simulink model "Full_model_M_function_spring_stiffness"  (R2018a)
settings: Solver=VariableStepAuto  StartTime=0.0  StopTime=10.0  FixedStep=0.00000001  RelTol=1e-3
values from neighbouring files (symbols this model uses):
  bs = 2000    [suspensiondata.mat]
  bse = 3000    [suspensiondata.mat]
  Kse = 8000    [suspensiondata.mat]
  Kt = 125000    [suspensiondata.mat]
  Ms = 250    [suspensiondata.mat]
  Mse = 90    [suspensiondata.mat]
  Mu = 40    [suspensiondata.mat]
  Zr = 0.2    [suspensiondata.mat]
undefined symbols (not defined in the file or in its folder): poly_coeffs, x_data, x_pivot, y_data, ypivot
settings Model: Creator=Saurabh Suman  LastModifiedBy=Saurabh Suman

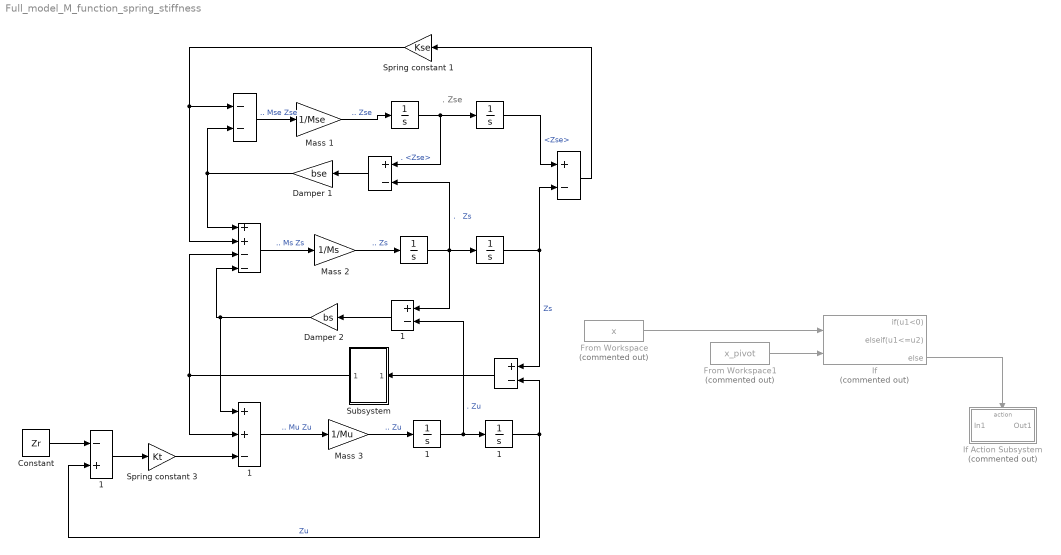
== system Full_model_M_function_spring_stiffness ==
  note: .
      | Zse
  " " : Integrator
  "  " : Sum  Inputs=+-
  "     " : Integrator
  "      " : Sum  Inputs=++--
  "       " : Sum  Inputs=--
  "        " : Sum  Inputs=+-
  "         " : Integrator
  "          " : Integrator
  "             " : Sum  Inputs=+-
  "             1" : Sum  Inputs=+-
  "          1" : Integrator
  "         1" : Integrator
  "       1" : Sum  Inputs=-+
  "      1" : Sum  Inputs=++-
  Constant : Constant  Value=Zr
  Damper 1 : Gain  Gain=bse
  Damper 2 : Gain  Gain=bs
  From Workspace : FromWorkspace  Commented=on  VariableName=x  SampleTime=0
  From Workspace1 : FromWorkspace  Commented=on  VariableName=x_pivot  SampleTime=0
  If : If  Commented=on  NumInputs=2  IfExpression=u1<0  ElseIfExpressions=u1<=u2
  If Action Subsystem : Subsystem  Commented=on  TreatAsAtomicUnit=on
  Mass 1 : Gain  Gain=1/Mse
  Mass 2 : Gain  Gain=1/Ms
  Mass 3 : Gain  Gain=1/Mu
  Spring constant 1 : Gain  Gain=Kse
  Spring constant 3 : Gain  Gain=Kt
  Subsystem : Subsystem
  wires:
  "     "/1 -> "  "/1  "<Zse>"
  "       1"/1 -> Spring constant 3/1
  " "/1 -> "        "/1, "     "/1  ". <Zse>"
  Mass 1/1 -> " "/1  ".. Zse"
  Damper 1/1 -> "      "/1, "       "/2
  Damper 2/1 -> "      "/4, "      1"/1
  Spring constant 3/1 -> "      1"/3
  "          "/1 -> "             "/1, "  "/2  "Zs"
  "      1"/1 -> Mass 3/1  ".. Mu Zu"
  "       "/1 -> Mass 1/1  ".. Mse Zse"
  Mass 3/1 -> "         1"/1  ".. Zu"
  "             1"/1 -> Damper 2/1
  "  "/1 -> Spring constant 1/1
  "         1"/1 -> "          1"/1, "             1"/2  ". Zu"
  "          1"/1 -> "       1"/2, "             "/2  "Zu"
  Constant/1 -> "       1"/1
  Spring constant 1/1 -> "      "/2, "       "/1
  "      "/1 -> Mass 2/1  ".. Ms Zs"
  Mass 2/1 -> "         "/1  ".. Zs"
  "         "/1 -> "        "/2, "          "/1, "             1"/1  ".   Zs"
  "        "/1 -> Damper 1/1
  From Workspace/1 -> If/1
  From Workspace1/1 -> If/2
  If/3 -> If Action Subsystem/Action
  Subsystem/1(Out1) -> "      "/3, "      1"/2
  "             "/1 -> Subsystem/1(In1)

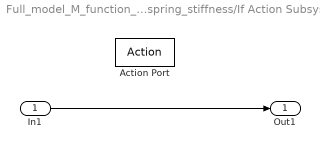
== system Full_model_M_function_spring_stiffness/If Action Subsystem ==
  In1 : Inport
  Action Port : ActionPort  ActionType=else
  Out1 : Outport
  wires:
  In1/1 -> Out1/1

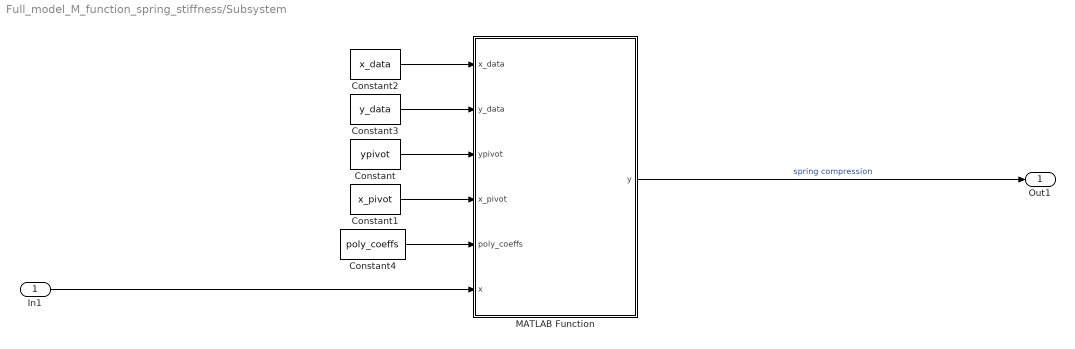
== system Full_model_M_function_spring_stiffness/Subsystem ==
  In1 : Inport
  Constant : Constant  Value=ypivot  VectorParams1D=off
  Constant1 : Constant  Value=x_pivot  VectorParams1D=off
  Constant2 : Constant  Value=x_data  VectorParams1D=off
  Constant3 : Constant  Value=y_data  VectorParams1D=off
  Constant4 : Constant  Value=poly_coeffs  VectorParams1D=off
  MATLAB Function : MATLAB Function  TreatAsAtomicUnit=on
  Out1 : Outport
  wires:
  MATLAB Function/1(y) -> Out1/1  "spring compression"
  In1/1 -> MATLAB Function/6(x)
  Constant4/1 -> MATLAB Function/5(poly_coeffs)
  Constant1/1 -> MATLAB Function/4(x_pivot)
  Constant3/1 -> MATLAB Function/2(y_data)
  Constant2/1 -> MATLAB Function/1(x_data)
  Constant/1 -> MATLAB Function/3(ypivot)

== matlab function Full_model_M_function_spring_stiffness/Subsystem/MATLAB Function ==
  data: x_data input; y_data input; ypivot input; x_pivot input; poly_coeffs input; x input; y output
function y = poly_limited(x_data, y_data, ypivot, x_pivot, poly_coeffs, x)
% Polynomial region
ypoly = polyval(poly_coeffs, x);
y1 = interp1(x_data, y_data, x_pivot);
y2 = interp1(x_data, y_data, x_pivot-0.01);
dfdx = (y2 -y1) / 0.01;

if x < 0
    y = 0;
elseif x <= x_pivot
    y = ypoly;
else
    y = ypivot + dfdx * (x - x_pivot);  % Linear extrapolation
end
